simulink model "PPS_Model"  (Simulink 7.6)
settings: Solver=FixedStepDiscrete  SolverMode=SingleTasking  StartTime=0.0  StopTime=inf  FixedStep=1/100  RelTol=1e-3
undefined symbols (not defined in the file): dfreq, gray, nbboxout, Rec, SDTV, strel
libraries: simulink x21, viptextngfix x15, simulink_extras x3, vipconversions x3, vipsnks x2, vipstatistics x1, dspmtrx3 x1, vipmorphops x1, vipanalysis x1
(part 2 of 2)

== system PPS_Model/PPS Model/Radar detection/TIS1 Sorting  Fun ==
  TIS1range [m] : Inport
  TIS1rangedot [m/s] : Inport  Port=2
  TIS1theta [deg] : Inport  Port=3
  Degrees to Radians : simulink_extras/Transformations/Degrees to Radians  SystemSampleTime=-1
  Switch : Switch  Criteria=u2 ~= 0
  Unary Minus : UnaryMinus
  Unary Minus1 : UnaryMinus
  range max : Constant  Value=TISMaxRange
  TIS1_RANGE [m] : Outport
  TIS1_RANGEDOT [m/s] : Outport  Port=2
  TIS1_THETA [rad] : Outport  Port=3
  wires:
  Unary Minus/1 -> Degrees to Radians/1
  Switch/1 -> TIS1_RANGE [m]/1
  TIS1rangedot [m/s]/1 -> Unary Minus1/1
  range max/1 -> Switch/3
  Degrees to Radians/1 -> TIS1_THETA [rad]/1
  TIS1range [m]/1 -> Switch/1, Switch/2
  TIS1theta [deg]/1 -> Unary Minus/1
  Unary Minus1/1 -> TIS1_RANGEDOT [m/s]/1

== system PPS_Model/PPS Model/Radar detection/Bend road segment/Lead Car Longitudinal Velocity1 ==
  TIS Rangedot [m/s] : Inport
  theta [rad] : Inport  Port=2
  lambda [rad] : Inport  Port=3
  Add1 : Sum  Inputs=+-
  Constant : Constant  Value=0
  Divide2 : Product  Inputs=*/
  Switch1 : Switch  Criteria=u2 ~= 0
  TIS1 Rangedot [m/s]1 : InportShadow  Port=1
  Trigonometric Function : Trigonometry  Operator=cos
  Vw [m/s] : Outport
  wires:
  TIS Rangedot [m/s]/1 -> Divide2/1
  lambda [rad]/1 -> Add1/1
  theta [rad]/1 -> Add1/2
  Add1/1 -> Trigonometric Function/1
  Trigonometric Function/1 -> Divide2/2
  Divide2/1 -> Switch1/1
  Switch1/1 -> Vw [m/s]/1
  TIS1 Rangedot [m/s]1/1 -> Switch1/2
  Constant/1 -> Switch1/3

== system PPS_Model/PPS Model/Radar detection/Bend road segment/Saturation1 ==
  TTCin : Inport
  TTCdem_in : Inport  Port=2  SampleTime=1/TISfreq
  Compare To Zero : simulink/Logic and Bit Operations/Compare To Zero  SystemSampleTime=-1  relop=<=  LogicOutDataTypeMode=uint8
  Gain : Gain  Gain=2
  Gain1 : Gain  Gain=ones(TISdet,1)
  Logical Operator : Logic  Operator=OR  AllPortsSameDT=off  OutDataTypeStr=boolean
  Relational Operator : RelationalOperator  Operator=>  OutDataTypeStr=boolean
  Switch : Switch  Criteria=u2 > Threshold  Threshold=0.5
  TTCout : Outport
  TTCdem_out : Outport  Port=2
  wires:
  Gain/1 -> Switch/1, Relational Operator/2
  Gain1/1 -> Gain/1, TTCdem_out/1
  Switch/1 -> TTCout/1
  TTCdem_in/1 -> Gain1/1
  Compare To Zero/1 -> Logical Operator/1
  Relational Operator/1 -> Logical Operator/2
  Logical Operator/1 -> Switch/2
  TTCin/1 -> Switch/3, Compare To Zero/1, Relational Operator/1

== system PPS_Model/PPS Model/Radar detection/Bend road segment/Saturation2 ==
  TTCin : Inport
  TTCdem_in : Inport  Port=2  SampleTime=1/TISfreq
  Compare To Zero : simulink/Logic and Bit Operations/Compare To Zero  SystemSampleTime=-1  relop=<=  LogicOutDataTypeMode=uint8
  Gain : Gain  Gain=2
  Gain1 : Gain  Gain=ones(TISdet,1)
  Logical Operator : Logic  Operator=OR  AllPortsSameDT=off  OutDataTypeStr=boolean
  Relational Operator : RelationalOperator  Operator=>  OutDataTypeStr=boolean
  Switch : Switch  Criteria=u2 > Threshold  Threshold=0.5
  TTCout : Outport
  TTCdem_out : Outport  Port=2
  wires:
  TTCin/1 -> Relational Operator/1, Compare To Zero/1, Switch/3
  Logical Operator/1 -> Switch/2
  Relational Operator/1 -> Logical Operator/2
  Compare To Zero/1 -> Logical Operator/1
  TTCdem_in/1 -> Gain1/1
  Switch/1 -> TTCout/1
  Gain1/1 -> TTCdem_out/1, Gain/1
  Gain/1 -> Relational Operator/2, Switch/1

== system PPS_Model/PPS Model/Radar detection/Bend road segment/Saturation3 ==
  TTCin : Inport
  TTCdem_in : Inport  Port=2  SampleTime=1/TISfreq
  Compare To Zero : simulink/Logic and Bit Operations/Compare To Zero  SystemSampleTime=-1  relop=<=  LogicOutDataTypeMode=uint8
  Gain : Gain  Gain=2
  Gain1 : Gain  Gain=ones(TISdet,1)
  Logical Operator : Logic  Operator=OR  AllPortsSameDT=off  OutDataTypeStr=boolean
  Relational Operator : RelationalOperator  Operator=>  OutDataTypeStr=boolean
  Switch : Switch  Criteria=u2 > Threshold  Threshold=0.5
  TTCout : Outport
  TTCdem_out : Outport  Port=2
  wires:
  TTCin/1 -> Relational Operator/1, Compare To Zero/1, Switch/3
  Logical Operator/1 -> Switch/2
  Relational Operator/1 -> Logical Operator/2
  Compare To Zero/1 -> Logical Operator/1
  TTCdem_in/1 -> Gain1/1
  Switch/1 -> TTCout/1
  Gain1/1 -> TTCdem_out/1, Gain/1
  Gain/1 -> Relational Operator/2, Switch/1

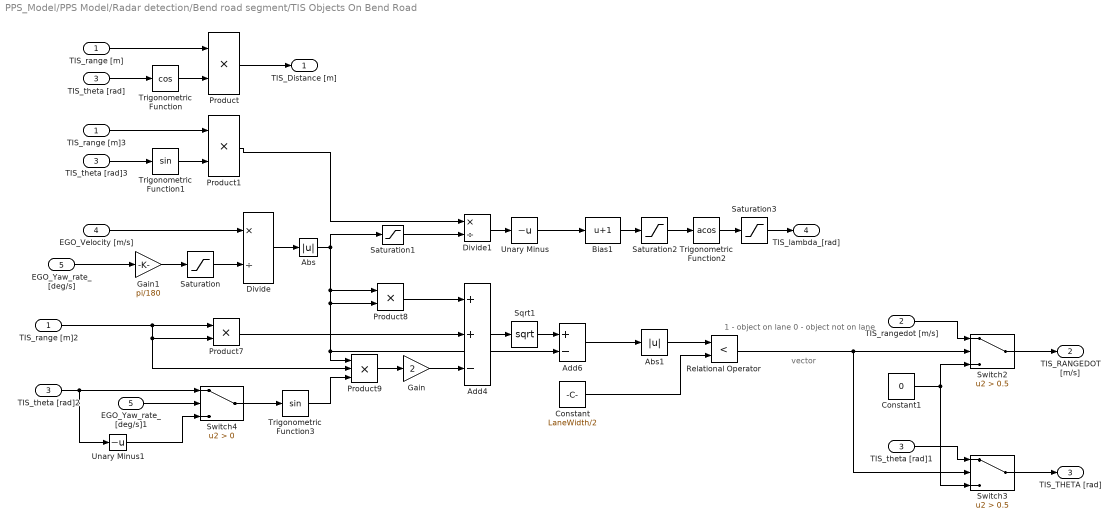
== system PPS_Model/PPS Model/Radar detection/Bend road segment/TIS Objects On Bend Road ==
  note: 1  - object      on lane
      | 0 - object not on lane
  note: vector
  TIS_range [m] : Inport
  TIS_rangedot [m/s] : Inport  Port=2
  TIS_theta [rad] : Inport  Port=3
  EGO_Velocity [m/s] : Inport  Port=4
  EGO_Yaw_rate_[deg/s] : Inport  Port=5
  Abs : Abs
  Abs1 : Abs
  Add4 : Sum  Inputs=++-
  Add6 : Sum  Inputs=+-
  Bias1 : Bias  Bias=1
  Constant : Constant  Value=LaneWidth/2
  Constant1 : Constant  Value=0
  Divide : Product  Inputs=*/
  Divide1 : Product  Inputs=*/
  EGO_Yaw_rate_[deg/s]1 : InportShadow  Port=5
  Gain : Gain  Gain=2
  Gain1 : Gain  Gain=pi/180
  Product{,1,7..8} (4 alike) : Product  RndMeth=Zero
  Product9 : Product  Inputs=3  RndMeth=Zero
  Relational Operator : RelationalOperator  Operator=<  OutDataTypeStr=boolean
  Saturation : Saturate  UpperLimit=inf  LowerLimit=1e-6
  Saturation1 : Saturate  UpperLimit=inf  LowerLimit=1e-6
  Saturation2 : Saturate  UpperLimit=1  LowerLimit=-1
  Saturation3 : Saturate  UpperLimit=pi  LowerLimit=0
  Sqrt1 : Math  Operator=sqrt  SaturateOnIntegerOverflow=on
  Switch2 : Switch  Criteria=u2 > Threshold  Threshold=0.5
  Switch3 : Switch  Criteria=u2 > Threshold  Threshold=0.5
  Switch4 : Switch  Criteria=u2 > Threshold
  TIS_range [m]2 : InportShadow  Port=1
  TIS_range [m]3 : InportShadow  Port=1
  TIS_theta [rad]1 : InportShadow  Port=3
  TIS_theta [rad]2 : InportShadow  Port=3
  TIS_theta [rad]3 : InportShadow  Port=3
  Trigonometric Function : Trigonometry  Operator=cos
  Trigonometric Function1 : Trigonometry
  Trigonometric Function2 : Trigonometry  Operator=acos
  Trigonometric Function3 : Trigonometry
  Unary Minus : UnaryMinus
  Unary Minus1 : UnaryMinus
  TIS_Distance [m] : Outport
  TIS_RANGEDOT [m/s] : Outport  Port=2
  TIS_THETA [rad] : Outport  Port=3
  TIS_lambda_[rad] : Outport  Port=4
  wires:
  TIS_range [m]/1 -> Product/1
  TIS_theta [rad]/1 -> Trigonometric Function/1
  Trigonometric Function/1 -> Product/2
  Trigonometric Function1/1 -> Product1/2
  EGO_Velocity [m/s]/1 -> Divide/1
  EGO_Yaw_rate_[deg/s]/1 -> Gain1/1
  Divide/1 -> Abs/1
  Relational Operator/1 -> Switch2/2, Switch3/2
  TIS_rangedot [m/s]/1 -> Switch2/1
  TIS_theta [rad]1/1 -> Switch3/1
  Constant1/1 -> Switch2/3, Switch3/3
  Switch2/1 -> TIS_RANGEDOT [m/s]/1
  Switch3/1 -> TIS_THETA [rad]/1
  Bias1/1 -> Saturation2/1
  Divide1/1 -> Unary Minus/1
  Unary Minus/1 -> Bias1/1
  Trigonometric Function2/1 -> Saturation3/1
  Abs/1 -> Product8/1, Product8/2, Product9/1, Add6/2, Saturation1/1
  Product/1 -> TIS_Distance [m]/1
  Product8/1 -> Add4/1
  Product7/1 -> Add4/2
  Gain/1 -> Add4/3
  Product9/1 -> Gain/1
  Trigonometric Function3/1 -> Product9/3
  Add4/1 -> Sqrt1/1
  Sqrt1/1 -> Add6/1
  Add6/1 -> Abs1/1
  EGO_Yaw_rate_[deg/s]1/1 -> Switch4/2
  Switch4/1 -> Trigonometric Function3/1
  TIS_theta [rad]2/1 -> Unary Minus1/1, Switch4/1
  TIS_range [m]2/1 -> Product7/1, Product7/2, Product9/2
  TIS_range [m]3/1 -> Product1/1
  TIS_theta [rad]3/1 -> Trigonometric Function1/1
  Product1/1 -> Divide1/1
  Abs1/1 -> Relational Operator/1
  Constant/1 -> Relational Operator/2
  Saturation/1 -> Divide/2
  Saturation1/1 -> Divide1/2
  Saturation2/1 -> Trigonometric Function2/1
  Saturation3/1 -> TIS_lambda_[rad]/1
  Gain1/1 -> Saturation/1
  Unary Minus1/1 -> Switch4/3

== system PPS_Model/PPS Model/Radar detection/Bend road segment/TTC Computing1 ==
  Distance [m] : Inport
  Velocity [m/s] : Inport  Port=2
  Compare : simulink/Logic and Bit Operations/Compare To Constant  SystemSampleTime=-1  relop===  const=1e-6  LogicOutDataTypeMode=uint8  ZeroCross=off
  Constant : Constant  Value=0
  Data Type Conversion : DataTypeConversion  OutDataTypeStr=double
  Product : Product  Inputs=*/  RndMeth=Zero
  Saturation : Saturate  UpperLimit=inf  LowerLimit=1e-6
  Switch : Switch  Criteria=u2 > Threshold
  Switch1 : Switch  Criteria=u2 > Threshold  Threshold=0.5
  TTC [s] : Outport
  wires:
  Velocity [m/s]/1 -> Switch/2, Switch/1
  Constant/1 -> Switch/3, Switch1/1
  Switch/1 -> Saturation/1
  Distance [m]/1 -> Product/1
  Saturation/1 -> Product/2, Compare/1
  Compare/1 -> Data Type Conversion/1
  Product/1 -> Switch1/3
  Switch1/1 -> TTC [s]/1
  Data Type Conversion/1 -> Switch1/2

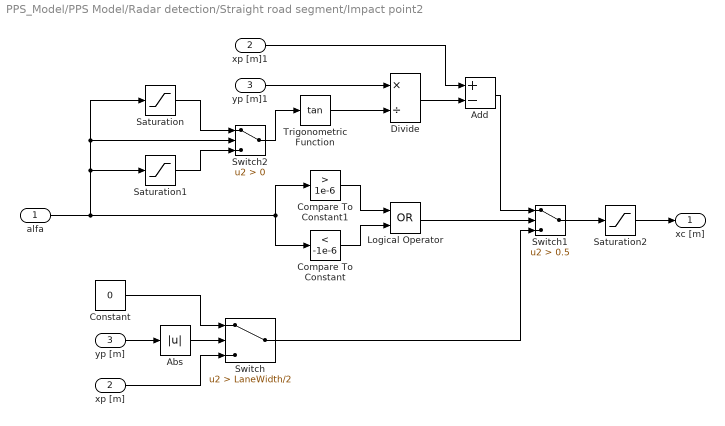
== system PPS_Model/PPS Model/Radar detection/Straight road segment/Impact point2 ==
  alfa : Inport
  xp [m] : Inport  Port=2
  yp [m] : Inport  Port=3
  Abs : Abs
  Add : Sum  Inputs=+-
  Compare To Constant : simulink/Logic and Bit Operations/Compare To Constant  SystemSampleTime=-1  relop=<  const=-1e-6  LogicOutDataTypeMode=uint8  ZeroCross=off
  Compare To Constant1 : simulink/Logic and Bit Operations/Compare To Constant  SystemSampleTime=-1  relop=>  const=1e-6  LogicOutDataTypeMode=uint8  ZeroCross=off
  Constant : Constant  Value=0
  Divide : Product  Inputs=*/
  Logical Operator : Logic  Operator=OR  AllPortsSameDT=off  OutDataTypeStr=boolean
  Saturation : Saturate  UpperLimit=inf  LowerLimit=1e-6
  Saturation1 : Saturate  UpperLimit=-1e-6  LowerLimit=-inf
  Saturation2 : Saturate  UpperLimit=300  LowerLimit=0
  Switch : Switch  Criteria=u2 > Threshold  Threshold=LaneWidth/2
  Switch1 : Switch  Criteria=u2 > Threshold  Threshold=0.5
  Switch2 : Switch  Criteria=u2 > Threshold
  Trigonometric Function : Trigonometry  Operator=tan
  xp [m]1 : InportShadow  Port=2
  yp [m]1 : InportShadow  Port=3
  xc [m] : Outport
  wires:
  yp [m]/1 -> Abs/1
  xp [m]/1 -> Switch/3
  Constant/1 -> Switch/1
  Switch/1 -> Switch1/3
  Abs/1 -> Switch/2
  xp [m]1/1 -> Add/1
  Divide/1 -> Add/2
  yp [m]1/1 -> Divide/1
  Trigonometric Function/1 -> Divide/2
  alfa/1 -> Compare To Constant1/1, Compare To Constant/1, Saturation1/1, Switch2/2, Saturation/1
  Compare To Constant1/1 -> Logical Operator/1
  Compare To Constant/1 -> Logical Operator/2
  Logical Operator/1 -> Switch1/2
  Switch1/1 -> Saturation2/1
  Add/1 -> Switch1/1
  Switch2/1 -> Trigonometric Function/1
  Saturation/1 -> Switch2/1
  Saturation1/1 -> Switch2/3
  Saturation2/1 -> xc [m]/1

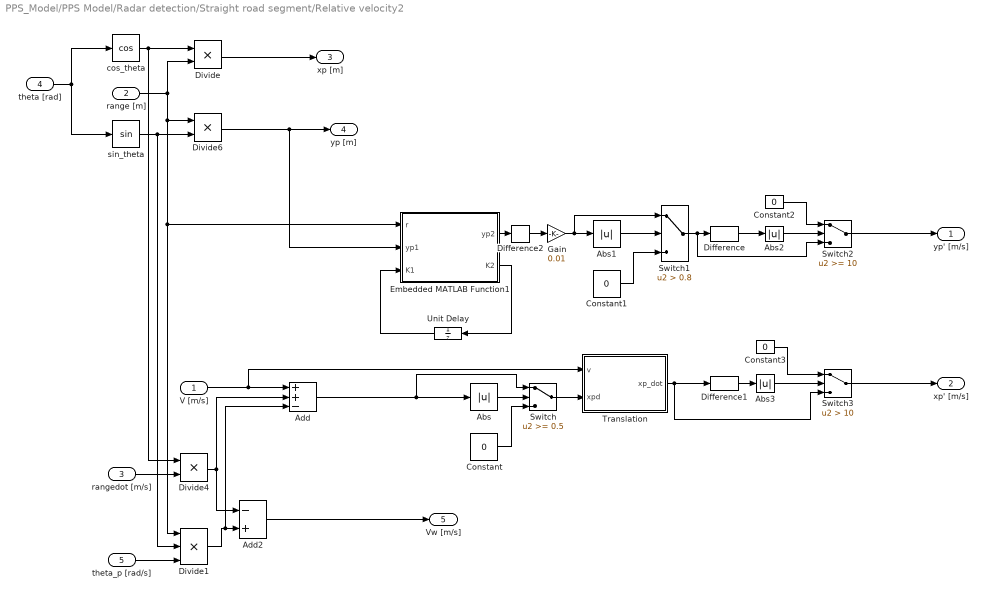
== system PPS_Model/PPS Model/Radar detection/Straight road segment/Relative velocity2 ==
  V [m/s] : Inport
  range [m] : Inport  Port=2
  rangedot [m/s] : Inport  Port=3
  theta [rad] : Inport  Port=4
  theta_p [rad/s] : Inport  Port=5
  Abs{,1..3} (4 alike) : Abs
  Add : Sum  Inputs=++-
  Add2 : Sum  Inputs=-+
  Constant{,1..3} (4 alike) : Constant  Value=0
  Difference : simulink/Discrete/Difference  SystemSampleTime=-1  ICPrevInput=zeros(TISdet,1)  OutMin=[]  OutMax=[]  OutDataType=fixdt(1, 16)  OutScaling=2^-10  DoSatur=off
  Difference1 : simulink/Discrete/Difference  SystemSampleTime=-1  ICPrevInput=zeros(TISdet,1)  OutMin=[]  OutMax=[]  OutDataType=fixdt(1, 16)  OutScaling=2^-10  DoSatur=off
  Difference2 : simulink/Discrete/Difference  SystemSampleTime=-1  ICPrevInput=0.0  OutMin=[]  OutMax=[]  OutDataType=sfix(16)  OutScaling=2^-10  DoSatur=off
  Divide : Product  Inputs=**
  Divide1 : Product  Inputs=***
  Divide4 : Product  Inputs=**
  Divide6 : Product  Inputs=**
  Embedded MATLAB Function1 : Stateflow chart  TreatAsAtomicUnit=on  SystemSampleTime=0.01
  Gain : Gain  Gain=0.01
  Switch : Switch  Threshold=0.5
  Switch1 : Switch  Criteria=u2 > Threshold  Threshold=0.8
  Switch2 : Switch  Threshold=10
  Switch3 : Switch  Criteria=u2 > Threshold  Threshold=10
  Translation : Stateflow chart  TreatAsAtomicUnit=on
  Unit Delay : UnitDelay  X0=zeros(TISdet,50)  SampleTime=-1
  cos_theta : Trigonometry  Operator=cos
  sin_theta : Trigonometry
  yp' [m/s] : Outport
  xp' [m/s] : Outport  Port=2
  xp [m] : Outport  Port=3
  yp [m] : Outport  Port=4
  Vw [m/s] : Outport  Port=5
  wires:
  rangedot [m/s]/1 -> Divide4/2
  Difference1/1 -> Abs3/1
  Constant3/1 -> Switch3/1
  Constant2/1 -> Switch2/1
  Switch3/1 -> xp' [m/s]/1
  Abs3/1 -> Switch3/2
  Translation/1(xp_dot) -> Difference1/1, Switch3/3
  Abs2/1 -> Switch2/2
  Difference/1 -> Abs2/1
  Switch2/1 -> yp' [m/s]/1
  Switch1/1 -> Switch2/3, Difference/1
  Constant1/1 -> Switch1/3
  Abs1/1 -> Switch1/2
  Gain/1 -> Switch1/1, Abs1/1
  Embedded MATLAB Function1/1(yp2) -> Difference2/1
  Unit Delay/1 -> Embedded MATLAB Function1/3(K1)
  Embedded MATLAB Function1/2(K2) -> Unit Delay/1
  Switch/1 -> Translation/2(xpd)
  Constant/1 -> Switch/3
  Abs/1 -> Switch/2
  Add/1 -> Switch/1, Abs/1
  V [m/s]/1 -> Translation/1(v), Add/1
  Divide1/1 -> Add/3, Add2/2
  Divide4/1 -> Add/2, Add2/1
  Add2/1 -> Vw [m/s]/1
  theta_p [rad/s]/1 -> Divide1/3
  Divide6/1 -> yp [m]/1, Embedded MATLAB Function1/2(yp1)
  cos_theta/1 -> Divide/1, Divide4/1
  sin_theta/1 -> Divide6/2, Divide1/2
  range [m]/1 -> Embedded MATLAB Function1/1(r), Divide1/1, Divide6/1, Divide/2
  Divide/1 -> xp [m]/1
  theta [rad]/1 -> cos_theta/1, sin_theta/1
  Difference2/1 -> Gain/1

== system PPS_Model/PPS Model/Radar detection/Straight road segment/Saturation1 ==
  TTCin : Inport
  TTCdem_in : Inport  Port=2  SampleTime=1/TISfreq
  Compare To Zero : simulink/Logic and Bit Operations/Compare To Zero  SystemSampleTime=-1  relop=<=  LogicOutDataTypeMode=uint8
  Gain : Gain  Gain=2
  Gain1 : Gain  Gain=ones(TISdet,1)
  Logical Operator : Logic  Operator=OR  AllPortsSameDT=off  OutDataTypeStr=boolean
  Relational Operator : RelationalOperator  Operator=>  OutDataTypeStr=boolean
  Switch : Switch  Criteria=u2 > Threshold  Threshold=0.5
  TTCout : Outport
  TTCdem_out : Outport  Port=2
  wires:
  Gain/1 -> Switch/1, Relational Operator/2
  Gain1/1 -> Gain/1, TTCdem_out/1
  Switch/1 -> TTCout/1
  TTCdem_in/1 -> Gain1/1
  Compare To Zero/1 -> Logical Operator/1
  Relational Operator/1 -> Logical Operator/2
  Logical Operator/1 -> Switch/2
  TTCin/1 -> Switch/3, Compare To Zero/1, Relational Operator/1

== system PPS_Model/PPS Model/Radar detection/Straight road segment/Saturation2 ==
  TTCin : Inport
  TTCdem_in : Inport  Port=2  SampleTime=1/TISfreq
  Compare To Zero : simulink/Logic and Bit Operations/Compare To Zero  SystemSampleTime=-1  relop=<=  LogicOutDataTypeMode=uint8
  Gain : Gain  Gain=2
  Gain1 : Gain  Gain=ones(TISdet,1)
  Logical Operator : Logic  Operator=OR  AllPortsSameDT=off  OutDataTypeStr=boolean
  Relational Operator : RelationalOperator  Operator=>  OutDataTypeStr=boolean
  Switch : Switch  Criteria=u2 > Threshold  Threshold=0.5
  TTCout : Outport
  TTCdem_out : Outport  Port=2
  wires:
  TTCin/1 -> Relational Operator/1, Compare To Zero/1, Switch/3
  Logical Operator/1 -> Switch/2
  Relational Operator/1 -> Logical Operator/2
  Compare To Zero/1 -> Logical Operator/1
  TTCdem_in/1 -> Gain1/1
  Switch/1 -> TTCout/1
  Gain1/1 -> TTCdem_out/1, Gain/1
  Gain/1 -> Relational Operator/2, Switch/1

== system PPS_Model/PPS Model/Radar detection/Straight road segment/Saturation3 ==
  TTCin : Inport
  TTCdem_in : Inport  Port=2  SampleTime=1/TISfreq
  Compare To Zero : simulink/Logic and Bit Operations/Compare To Zero  SystemSampleTime=-1  relop=<=  LogicOutDataTypeMode=uint8
  Gain : Gain  Gain=2
  Gain1 : Gain  Gain=ones(TISdet,1)
  Logical Operator : Logic  Operator=OR  AllPortsSameDT=off  OutDataTypeStr=boolean
  Relational Operator : RelationalOperator  Operator=>  OutDataTypeStr=boolean
  Switch : Switch  Criteria=u2 > Threshold  Threshold=0.5
  TTCout : Outport
  TTCdem_out : Outport  Port=2
  wires:
  TTCin/1 -> Relational Operator/1, Compare To Zero/1, Switch/3
  Logical Operator/1 -> Switch/2
  Relational Operator/1 -> Logical Operator/2
  Compare To Zero/1 -> Logical Operator/1
  TTCdem_in/1 -> Gain1/1
  Switch/1 -> TTCout/1
  Gain1/1 -> TTCdem_out/1, Gain/1
  Gain/1 -> Relational Operator/2, Switch/1

== system PPS_Model/PPS Model/Radar detection/Straight road segment/THETA Derivative1 ==
  range [m] : Inport
  theta [rad] : Inport  Port=2
  Abs1 : Abs
  Deriv correction : Stateflow chart  TreatAsAtomicUnit=on
  Difference1 : simulink/Discrete/Difference  SystemSampleTime=-1  ICPrevInput=0.0  OutMin=[]  OutMax=[]  OutDataType=sfix(16)  OutScaling=2^-10  DoSatur=off
  Difference2 : simulink/Discrete/Difference  SystemSampleTime=-1  ICPrevInput=0.0  OutMin=[]  OutMax=[]  OutDataType=sfix(16)  OutScaling=2^-10  DoSatur=off
  Digital Clock : DigitalClock  SampleTime=1/TISfreq
  Gain : Gain  Gain=0.01
  Gain1 : Gain  Gain=0.01
  Memory : Memory  X0=zeros(TISdet,10,2)  InheritSampleTime=on
  Memory1 : Memory  X0=zeros(TISdet,1)  InheritSampleTime=on
  Memory2 : Memory  X0=zeros(TISdet,1)  InheritSampleTime=on
  Switch : Switch  Threshold=2
  Theta extrapolation : Stateflow chart  TreatAsAtomicUnit=on
  theta_dot [rad/s] : Outport
  wires:
  Memory1/1 -> Deriv correction/2(thp)
  Gain1/1 -> Deriv correction/3(thd)
  Theta extrapolation/1(th2) -> Deriv correction/1(th), Memory1/1, Difference1/1
  range [m]/1 -> Theta extrapolation/1(r)
  Gain/1 -> Theta extrapolation/3(thd)
  Digital Clock/1 -> Theta extrapolation/4(time)
  Memory/1 -> Theta extrapolation/5(K1)
  Theta extrapolation/2(K2) -> Memory/1
  theta [rad]/1 -> Theta extrapolation/2(th1), Difference2/1
  Deriv correction/1(th_dot) -> Switch/3, Abs1/1
  Switch/1 -> Memory2/1, theta_dot [rad/s]/1
  Abs1/1 -> Switch/2
  Memory2/1 -> Switch/1
  Difference2/1 -> Gain/1
  Difference1/1 -> Gain1/1

== system PPS_Model/PPS Model/Radar detection/Straight road segment/TTC computing1 ==
  xc [m] : Inport
  Vw [m/s] : Inport  Port=2
  Compare To Constant : simulink/Logic and Bit Operations/Compare To Constant  SystemSampleTime=-1  relop===  const=1e-6  LogicOutDataTypeMode=uint8  ZeroCross=off
  Constant : Constant  Value=0
  Data Type Conversion : DataTypeConversion  OutDataTypeStr=double
  Divide : Product  Inputs=/*
  Saturation : Saturate  UpperLimit=inf  LowerLimit=1e-6
  Switch : Switch  Criteria=u2 > Threshold
  Switch1 : Switch  Criteria=u2 > Threshold  Threshold=0.5
  TTC : Outport  InitialOutput=0
  wires:
  Vw [m/s]/1 -> Switch/2, Switch/1
  Constant/1 -> Switch/3, Switch1/1
  Switch/1 -> Saturation/1
  Saturation/1 -> Divide/1, Compare To Constant/1
  Compare To Constant/1 -> Data Type Conversion/1
  xc [m]/1 -> Divide/2
  Divide/1 -> Switch1/3
  Switch1/1 -> TTC/1
  Data Type Conversion/1 -> Switch1/2

== system PPS_Model/PPS Model/Radar detection/Straight road segment/alfa1 ==
  yp'1 : Inport
  xp' : Inport  Port=2
  Abs : Abs
  Compare To Constant : simulink/Logic and Bit Operations/Compare To Constant  SystemSampleTime=-1  relop===  const=pi/2  LogicOutDataTypeMode=uint8
  Constant : Constant  Value=0
  Switch : Switch  Criteria=u2 > Threshold
  four quadrant atan : Trigonometry  Operator=atan2
  alfa1 : Outport
  wires:
  yp'1/1 -> four quadrant atan/1
  xp'/1 -> four quadrant atan/2
  four quadrant atan/1 -> Abs/1, Switch/3
  Abs/1 -> Compare To Constant/1
  Compare To Constant/1 -> Switch/2
  Constant/1 -> Switch/1
  Switch/1 -> alfa1/1

== matlab function PPS Model/Radar detection/Straight road segment/Relative velocity2/Embedded MATLAB Function1 ==
  data: r input double; yp2 output double; yp1 input double; K1 input double; K2 output double; TISdet parameter double; TISMaxRange parameter double
function [yp2, K2] = modif(r, yp1, K1, TISdet, TISMaxRange)
%#eml
% Interpolating yp value.

K2 = K1;
yp2 = yp1;

d = 50;

% Adding point
for i = 1 : TISdet
   if r(i) ~= 150
      K2(i,1:d-1) = K2(i,2:d);
      K2(i,d) = yp1(i);
   end
end

% Choosing what to take
for i = 1 : TISdet
    s = 0;
    suma = 0;
    for j = 1 : 50
        if K2(i,j) ~= 0
            suma = suma + K2(i,j);
            s = s + 1;
        end
    end
    yp2(i) = suma/s;
end

% Returning, if object is not detected
for i = 1: TISdet
    if r(i) == TISMaxRange && yp1(i) == 0
        K2(i,:,:) = zeros(d,1);
        yp2(i) = 0;
    end    
end

== matlab function PPS Model/Radar detection/Straight road segment/Relative velocity2/Translation ==
  data: v input double; xpd input double; xp_dot output double; TISdet parameter double
function xp_dot = trans(v, xpd, TISdet)
%#codegen
%Translation of the value

xp_dot = xpd;
for i = 1 : TISdet
    if xpd(i) == v
        xp_dot(i) =0;
    end
end
end

== matlab function PPS Model/Pedestrian detection/POSITION ==
  data: flag input double size=TISdet; theta input double size=TISdet; posit output double; range input double; xs_m output double; ys_m output double; TISdet parameter double; TISMaxRange parameter double
function [posit,xs_m,ys_m]= positt(flag,theta,range,TISdet, TISMaxRange)
%#codegen
xposit = zeros(1,TISdet);
yposit = zeros(1,TISdet);
posit = zeros(2,TISdet);
xs_m = zeros(1,TISdet);
ys_m = zeros(1,TISdet);
X_offset = 3.9 - 1.9;                                   %Offset Between Camera and Radar Positions
Z_offset = 0.42 - 1.28;                                 %Offset Between Camera and Radar Positions

f = 0.0075;                                             %Focal Length
sx = 0.0048;                                            %Pixel Width
%Maximum Camera Cooridnates%
u_max = TISMaxRange * sin(23.1*pi/180);                          %radar range = 40m, camera fov = 46.2 degrees 
v_max = TISMaxRange * cos(23.1*pi/180);

for i=1:TISdet
    if (flag(i)==0) || (theta(i)==0)
        xposit(i) = 0;
        posit(1,i) = 0;
    elseif (flag(i)~=0)
        theta_aux = -theta(i);      
        
        X = range(i)*cos(theta_aux*pi/180);
        Y = range(i)*sin(theta_aux*pi/180);
        
        xs_m(i) = Y;        
        ys_m(i) = X;
        %Camera 3-D Coordinates%
        X_c = X + X_offset;
        Y_c = Y;

        %Camera Pixel Coordinates%
        u_r_new = (Y*f*500)/(sx*u_max);
      
        %Conversion of xc to pixel value%
        xposit(i)= 250 + u_r_new;
        yposit(i)=188;
    end
     posit(2,i)=round(xposit(i));
     posit(1,i)=round(yposit(i));
end

== matlab function PPS Model/Pedestrian detection/scaling_crop ==
  data: im input double; PosObj input double; X input double; Y input double; sub_im output double size=[375 500]; posObj_subim output double; im_x output double; im_y output double; liminf_x output double; liminf_y output double; rectangle output double
function [sub_im,posObj_subim,im_x,im_y,liminf_x, liminf_y,rectangle]=escaling(im,PosObj,X,Y)

minPx=size(im,2);
minPy=size(im,1);
maxPx=0;
maxPy=0;
detected=0;
mino=0;
maxo=0;
for i=1:size(PosObj,2)
    if PosObj(2,i)~=0
        if(PosObj(2,i)<minPx)
            minPx=PosObj(2,i);
            minPy=PosObj(1,i);
            mino=i;
        end
        if (PosObj(2,i)>maxPx)
            maxPx=PosObj(2,i);
            maxPy=PosObj(1,i);
            maxo=i;
        end
        detected=detected+1;
    end
end
if (detected==0)
    liminf_x=size(im,2);
    limsup_x=size(im,2);
    liminf_y=size(im,1);
    limsup_y=size(im,1);
 
 else
   
  %%For horizontal and vertical position
   
  if (mino~=0) 
    liminf_x= round(minPx-((40-round(1.6*Y(mino)))*2));
    liminf_y= round(minPy-((100-round(4.5*Y(mino)))*2));
    
  else
     liminf_x=1;
     liminf_y=1;
  end
   if (maxo~=0)   
    limsup_x= abs(round(maxPx+((40-round(1.6*Y(maxo)))*2)));
    limsup_y= abs(round(maxPy+((100-round(5*Y(maxo)))*2)));
   else
       limsup_x=size(im,2);
       limsup_y=size(im,1);
   end

end

  if (liminf_x<1)
         liminf_x=1;
  end
    
  if (limsup_x>size(im,2))
        limsup_x=size(im,2);
  end
    
  if (liminf_y<1)
       liminf_y=1;
  end
    
  if (limsup_y>=size(im,1))
       limsup_y=size(im,1);
  end
  
  if (liminf_y > size(im,1))
        liminf_y = size(im,1);
  end
    
   posObj_subim=zeros(2,size(PosObj,2));
   a=1;
    
    for i=1:size(PosObj,2)
        if (PosObj(2,i)~=0)
            posObj_subim(:,a)=[PosObj(1,i)-liminf_y;PosObj(2,i)-liminf_x];
            a=a+1;
        end
    end

sub_im=im(liminf_y:limsup_y,liminf_x:limsup_x);

if length( sub_im ) < 3
    sub_im = zeros(3,3,'uint8');
end


im_x=limsup_x-liminf_x;
im_y=limsup_y-liminf_y;
rectangle=[liminf_y liminf_x im_y im_x];

== matlab function PPS Model/Radar detection/Straight road segment/THETA Derivative1/Deriv correction ==
  data: th input double; thp input double; thd input double; th_dot output double; TISdet parameter double
function th_dot = stopping(th, thp, thd, TISdet)
%#codegen
% Stopping if nothing is detected.

th_dot = thd;
for i = 1 : TISdet
    if (th(i)==0 && thp(i)~=0) || (th(i)~=0 && thp(i)==0)
        th_dot(i) = 0;
    end
end
end

== matlab function PPS Model/Radar detection/Straight road segment/THETA Derivative1/Theta extrapolation ==
  data: r input double; th1 input double; th2 output double; thd input double; time input double; K1 input double; K2 output double; TISdet parameter double; TISMaxRange parameter double
function [th2, K2] = modif(r, th1, thd, time, K1, TISdet, TISMaxRange)
%#codegen
% Interpolating theta value.

K2 = K1;
th2 = th1;

d = 10;

% Finding points used in interpolation/extrapolation.
for i = 1 : TISdet
    if thd(i) ~= 0
        K2(i,1:d-1,:) = K2(i,2:d,:);
        K2(i,  d,1) = time;
        K2(i,  d,2) = th1(i);
    end
end

% Extrapolation
for i = 1 : TISdet
    j = 1;
    while j < d+1 && K2(i,j,1) == 0
        j = j + 1;
    end
    
    if j > d-2
        th2(i) = th1(i);
    else
        th2(i) = interp1(K2(i,d-2:d,1),K2(i,d-2:d,2),time,'linear','extrap');
    end
end

% Returning, if object is not detected
for i = 1: TISdet
    if r(i) == TISMaxRange && th1(i) == 0
        K2(i,:,:) = zeros(d,2);
        th2(i) = 0;
    end    
end

end

== matlab function PPS Model/Pedestrian detection/Blob Analysis/Embedded MATLAB Function1 ==
  data: centroid input double; centout output double; bbox input double; bboxout output double; majoraxis input double; minoraxis input double; orientation input double; eccentricity input double; label input double; label_out output double size=[400 550]; im_x input double; im_y input double; posObj_subim input double; liminf_x input double; liminf_y input double; posObj_im output double
function [centout,bboxout,label_out,posObj_im] = select_blobs(centroid,bbox,majoraxis,minoraxis,orientation,eccentricity,label,im_x,im_y,posObj_subim, liminf_x,liminf_y)
%#eml
a=1;
centroid=int32(centroid);
centout=int32(zeros(2,size(centroid,2)));
bboxout=int32(zeros(4,size(bbox,2)));
label_out=zeros(size(label,1),size(label,2));
posObj_im=posObj_subim;
for i=1:size(posObj_subim,2)
    posObj_im(:,i)=posObj_subim(:,i)+[liminf_y;liminf_x];
end

for i=1:size(orientation,2)
    touch=0;
    if orientation(1,i)>=180
         or_val=360-orientation(1,i);
     else
         or_val=orientation(1,i);
     end
     lr=bbox(1,i)+1;
     lh=lr+bbox(3,i)-1;
     lc=bbox(2,i)+1;
     lw=lc+bbox(4,i)-1;
      if (bbox(1,i)==0)
          touch=touch+1;
      end
      if (bbox(2,i)==0)
          touch=touch+1;
      end
      if(im_y-centroid(1,i)-(bbox(4,i)/2)<2)
          touch=touch+1;
      end
      if (im_x-centroid(2,i)-(bbox(3,i)/2)<2)
          touch=touch+1;
      end
     
     if (abs(or_val)>55)&&(abs(or_val)<145)&&((majoraxis(i)/minoraxis(i))>1.5)&&((majoraxis(i)/minoraxis(i))<3)&&(eccentricity(i)>0)&&(eccentricity(i)<1)&&(touch<2)
         bboxout(1:2,a)= bbox(1:2,i)+int32([liminf_y;liminf_x]);
         bboxout(3:4,a)= bbox(3:4,i);
         centout(:,a)= centroid(:,i)+int32([liminf_y;liminf_x]);
         label_out(lr:lh,lc:lw)=a;
         a=a+1;
     else
        label_out(lr:lh,lc:lw)=0;
     end
end

== matlab function PPS Model/Pedestrian detection/Blob Analysis/Embedded MATLAB Function2 ==
  data: nbboxout input double; label input double; r_label output double; color output double
function [r_label,color] = r_labels(nbboxout,label)
%#eml
n=size(nbboxout,2);
r_label=zeros(1,n);
color=zeros(1,n);
not_before=1;
a=1;
for i=1:size(label,1)
    for j=1:size(label,2)
        if (a==1)
            if (label(i,j)~=0)
                r_label(1,a)=label(i,j);
                a=a+1;
            end
        else
             if (label(i,j)~=0)
                 for h=1:a
                     if(label(i,j)~=r_label(1,h))
                         not_before=1;
                     else
                         not_before=0;
                         break
                     end
                 end
                 if not_before==1
                     r_label(1,a)=label(i,j);
                     a=a+1;
                 end
             end
        end 
    end 
end
color(1,:)=2;

== matlab function PPS Model/Pedestrian detection/Image processing/Embedded MATLAB Function ==
  data: im output double size=[375 500]; image input double
function im = sub_image(image)
%#eml
im=zeros(size(image,1),size(image,2));
for i=1:size(image,1)
    for j=1:size(image,2)
        if (image(i,j)==0)
            im(i,j)=1;
        else
            im(i,j)=0;
        end
    end
end

== matlab function PPS Model/Pedestrian detection/PEDES ==
  data: CentAlarms output double; PosObj_subim input double; Centroid_subim input double; alarms output double size=TISdet; BBox input double; BBox_det output double; TISdet parameter double
function [CentAlarms,alarms,BBox_det]= pedes(PosObj_subim, Centroid_subim,BBox,TISdet)
%#eml
CentAlarms=int32(zeros(2,size(PosObj_subim,2)));
alarms=zeros(size(PosObj_subim,2),1);
BBox_det=int32(zeros(4,size(BBox,2)));
a=1;
for i=1:size(PosObj_subim,2)
    for j=1:size(Centroid_subim,2)
        if (Centroid_subim(1,j)~=0)||(Centroid_subim(2,j)~=0)
            if (abs(Centroid_subim(2,j)-PosObj_subim(2,i))<15)||(abs(Centroid_subim(1,j)-PosObj_subim(1,i))<15)%(PosObj_subim(1,i))>BBox(1,j)&&(PosObj_subim(1,i))<(BBox(1,j)+BBox(3,j))
                alarms(a,1)=1;
                CentAlarms(:,a)=PosObj_subim(:,i);%Centroid_subim(:,j);
                BBox_det(:,a)=BBox(:,i);
            end
        end
    end
    a=a+1;
end

== matlab function PPS Model/Pedestrian detection/PEDES1 ==
  data: Im input double size=[375 500]; Imout output double size=[375 500 3]
function Imout = imag(Im)
%#eml
Imout=128*ones(size(Im,1),size(Im,2),3);
Imout(:,:,1)=Im;

== matlab function PPS Model/Pedestrian detection/PEDES2 ==
  data: Im input double size=[375 500]; Imout output double size=[375 500 3]
function Imout = imag(Im)
%#eml
Imout=128*ones(size(Im,1),size(Im,2),3);
Imout(:,:,1)=Im;

== matlab function PPS Model/Pedestrian detection/PEDES3 ==
  data: inpoints output double; pts input double
function inpoints= points(pts)
%#eml
inpoints = pts;
for i=1:size(pts,1)
    for j=1:2
         inpoints(i,j)=pts(i,j)+1;
    end
     for j=3:4
         inpoints(i,j)=pts(i,j)-1;
    end
end

== matlab function PPS Model/Pedestrian detection/PEDES5 ==
  data: blob_subim_proces output double; sub_im input double size=[375 500]; limx_inf input double; limy_inf input double; im_x input double; im_y input double
function blob_subim_proces = blob_subim(sub_im, limx_inf, limy_inf,im_x,im_y)
%#eml
blob_subim_proces=single(zeros(375,500));

limx_sup=limx_inf+im_x;
limy_sup=limy_inf+im_y;

% Assigned the superior and inferior limit 
limx_sup_sorted=max([limx_sup limx_inf]);
limx_inf_sorted=min([limx_sup limx_inf]);
limy_inf_sorted=min([limy_sup limy_inf]);
limy_sup_sorted=max([limy_sup limy_inf]);


[nn, mm] = size( sub_im );
if ( nn <= 3 ) && ( mm <= 3 )
    sub_im = 0;
    % Create a zeros matrix of size (im_y,im_x)
    if im_x~=0 || im_y~=0
        im_x=abs(im_x);
        im_y=abs(im_y);
        assert(im_x<1000);
        assert(im_y<1000);
        sub_im=zeros(im_y+1,im_x+1);
    end
end


blob_subim_proces(limy_inf_sorted:limy_sup_sorted,limx_inf_sorted:limx_sup_sorted)=sub_im;
